simulink model "cantonisim_distributed_3pools"  (R2019b)
settings: Solver=VariableStepAuto  StartTime=0.0  StopTime=800  FixedStep=1  RelTol=1e-3
InitFcn:
  | ini_cantonisim_distributed
values from neighbouring files (symbols this model uses):
  alpha = [6492, 2478, 6084, 5658, 7650, 6492]    [cantoni_2008_values.m]    (also in cantoni_LMI.m = [6492, 2478, 6084, 5658, 7650]; distributed_workspace.mat = [6492 2478 6084 5658 7650])
  kappa = [1.69, 6.47, 2.37, 2.21, 1.68, 1.69]    [cantoni_2008_values.m]    (also in cantoni_LMI.m = [1.69, 6.47, 2.37, 2.21, 1.68]; distributed_workspace.mat = [1.69 6.47 2.37 2.21 1.68]; lab_setup_values.m = [0.3, 0.5, 0.3])
  phi = [113.64, 37.17, 86.96, 96.15, 113.64, 113.64]    [cantoni_2008_values.m]    (also in cantoni_LMI.m = [113.64, 37.17, 86.96, 96.15, 113.64]; distributed_workspace.mat = [113.64 37.17 86.96 96.15 113.64]; lab_setup_values.m = [10, 10, 10])
  rho = [9.97, 3.26, 7.60, 8.47, 9.97, 9.97]    [cantoni_2008_values.m]    (also in cantoni_LMI.m = [9.97, 3.26, 7.60, 8.47, 9.97]; distributed_workspace.mat = [9.97 3.26 7.6 8.47 9.97]; lab_setup_values.m = [0.1, 0.1, 0.1])
  tau = [4, 2, 4, 4, 6, 4]    [cantoni_2008_values.m]    (also in cantoni_LMI.m = [4, 2, 4, 4, 6]; distributed_workspace.mat = [4 2 4 4 6])
  w_n = zeros(1,length(phi_wave))    [cantoni_2008_values.m]    (also in cantoni_LMI.m; distributed_workspace.mat = [0.48005473176 1.05011972572 0.48005473176 0.48005473176 0.4)
  zeta = 0.0151    [distributed_workspace.mat]
undefined symbols (not defined in the file or in its folder): SA, SB, SC, SD
settings Model: Creator=Jacob  LastModifiedBy=bas
settings SolverCC: AlgebraicLoopSolver=LineSearch
settings ModelReferenceCC: ModelReferenceMinAlgLoopOccurrences=on
settings SFSimCC: CustomCodeUndefinedFunction=UseInterfaceOnly

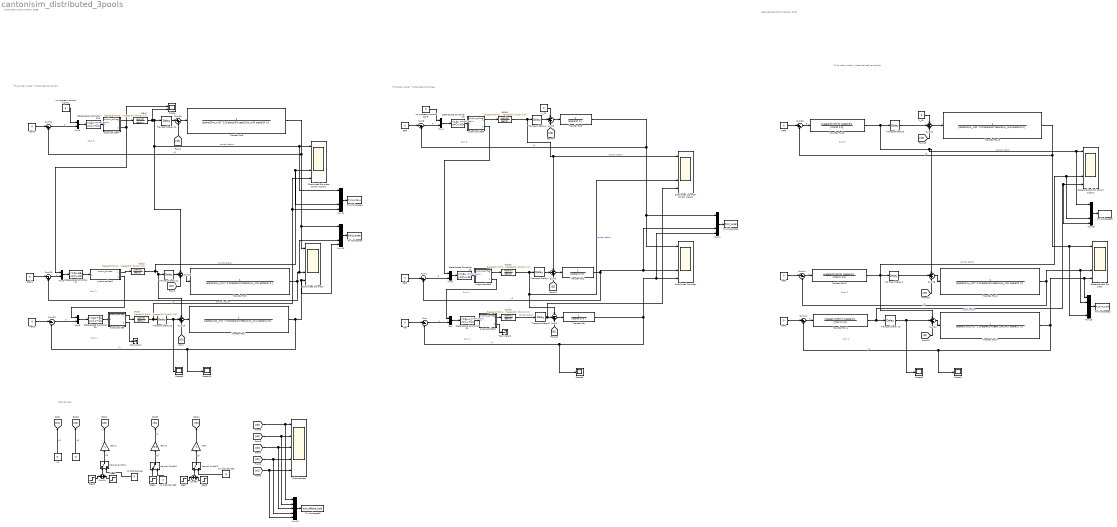
== system cantonisim_distributed_3pools ==
  note: Disturbances
  note: Decentralied Control Cantoni 2007
  note: Third order model + decentralized controllers
  note: First order model + distributed controllers
  note: Pool 1
  note: Distributed Control Cantoni 2008
  note: Pool 2
  note: Pool 5
  note: Pool 1
  note: Pool 5
  note: Pool 2
  note: Third order model + distributed controllers
  note: Pool 5
  note: Pool 1
  note: Pool 2
  " " : Constant  Value=0
  Decentralized 3rd control signals : Scope  NumInputPorts=5
  Decentralized 3rd order : Scope  NumInputPorts=5
  Distributed 1st order : Scope  NumInputPorts=5
  Distributed 1st order control signals : Scope  NumInputPorts=5
  Distributed 3rd order : Scope  NumInputPorts=5
  Distributed 3rd order control signals : Scope  NumInputPorts=5
  Disturbances : Scope  NumInputPorts=5
  Gain : Gain  Gain=-1
  Gain1 : Gain  Gain=-1
  Gain2 : Gain  Gain=-0.5
  Manual Switch1 : ManualSwitch
  Manual Switch2 : ManualSwitch
  Manual Switch3 : ManualSwitch
  Mux{,1,4..6,9} (6 alike) : Mux  Inputs=2
  Mux{10..15} (6 alike) : Mux  Inputs=5
  Ref{,1,4..6,9..11,14} (9 alike) : Constant  Value=0
  Scope : Scope  NumInputPorts=2
  Scope{3,5,7..8,10} (5 alike) : Scope
  State-Space Controller S1 : StateSpace  A=SA{1}  B=SB{1}  C=SC{1}  D=SD{1}  InitialCondition=0
  State-Space Controller S10 : StateSpace  A=SA{3}  B=SB{3}  C=SC{3}  D=SD{3}  InitialCondition=0
  State-Space Controller S2 : StateSpace  A=SA{2}  B=SB{2}  C=SC{2}  D=SD{2}  InitialCondition=0
  State-Space Controller S5 : StateSpace  A=SA{3}  B=SB{3}  C=SC{3}  D=SD{3}  InitialCondition=0
  State-Space Controller S6 : StateSpace  A=SA{1}  B=SB{1}  C=SC{1}  D=SD{1}  InitialCondition=0
  State-Space Controller S7 : StateSpace  A=SA{2}  B=SB{2}  C=SC{2}  D=SD{2}  InitialCondition=0
  Step1 : Step  Time=100  SampleTime=0
  Step5 : Step  Time=10  SampleTime=0
  Step6 : Step  Time=20  After=-1  SampleTime=0
  Step7 : Step  Time=100  SampleTime=0
  Step8 : Step  Time=150  After=-1  SampleTime=0
  Sum{,10,14,20} (4 alike) : Sum  Inputs=|+-
  Sum{1,3,9,12,15,21,23,26} (8 alike) : Sum  Inputs=-++
  Sum{2,8,25,31} (4 alike) : Sum  Inputs=|-+
  Sum22 : Sum  Inputs=|--
  Sum24 : Sum  Inputs=+|+
  Sum32 : Sum  Inputs=|++
  Sum33 : Sum  Inputs=+|+
  Terminator : Terminator
  Terminator1 : Terminator
  To Workspace : ToWorkspace  VariableName=third_order  SaveFormat=Structure With Time  SampleTime=-1
  To Workspace1 : ToWorkspace  VariableName=first_order  SaveFormat=Structure With Time  SampleTime=-1
  To Workspace2 : ToWorkspace  VariableName=dist_offtake_load  SaveFormat=Structure With Time  SampleTime=-1
  To Workspace3 : ToWorkspace  VariableName=PI_third_order  SaveFormat=Structure With Time  SampleTime=-1
  To Workspace4 : ToWorkspace  VariableName=third_order_u  SaveFormat=Structure With Time  SampleTime=-1
  To Workspace5 : ToWorkspace  VariableName=PI_third_order_u  SaveFormat=Structure With Time  SampleTime=-1
  Transfer Fcn : TransferFcn  Denominator=[alpha(1) 0 ]
  Transfer Fcn1 : TransferFcn  Denominator=[alpha(1)/w_n(1)^2 2*alpha(1)*zeta(1)/w_n(1) alpha(1) 0 ]
  Transfer Fcn10 : TransferFcn  Denominator=[alpha(1)/w_n(1)^2 2*alpha(1)*zeta(1)/w_n(1) alpha(1) 0 ]
  Transfer Fcn11 : TransferFcn  Numerator=[kappa(1)*phi(1) kappa(1)]  Denominator=[rho(1) 1 0]
  Transfer Fcn12 : TransferFcn  Denominator=[alpha(2)/w_n(2)^2 2*alpha(2)*zeta(2)/w_n(2) alpha(2) 0 ]
  Transfer Fcn13 : TransferFcn  Numerator=[kappa(2)*phi(2) kappa(2)]  Denominator=[rho(2) 1 0]
  Transfer Fcn18 : TransferFcn  Denominator=[alpha(3)/w_n(3)^2 2*alpha(3)*zeta(3)/w_n(3) alpha(3) 0 ]
  Transfer Fcn19 : TransferFcn  Numerator=[kappa(3)*phi(3) kappa(3)]  Denominator=[rho(3) 1 0]
  Transfer Fcn2 : TransferFcn  Denominator=[alpha(2) 0 ]
  Transfer Fcn3 : TransferFcn  Denominator=[alpha(2)/w_n(2)^2 2*alpha(2)*zeta(2)/w_n(2) alpha(2) 0 ]
  Transfer Fcn8 : TransferFcn  Denominator=[alpha(3) 0 ]
  Transfer Fcn9 : TransferFcn  Denominator=[alpha(3)/w_n(3)^2 2*alpha(3)*zeta(3)/w_n(3) alpha(3) 0 ]
  Transport Delay1 : TransportDelay  DelayTime=tau(2)
  Transport Delay10 : TransportDelay  DelayTime=tau(1)
  Transport Delay11 : TransportDelay  DelayTime=tau(2)
  Transport Delay14 : TransportDelay  DelayTime=tau(3)
  Transport Delay15 : TransportDelay  DelayTime=tau(1)
  Transport Delay4 : TransportDelay  DelayTime=tau(3)
  Transport Delay5 : TransportDelay  DelayTime=tau(1)
  Transport Delay6 : TransportDelay  DelayTime=tau(2)
  Transport Delay9 : TransportDelay  DelayTime=tau(3)
  V_N1 : Constant  Value=0
  V_N2 : Constant  Value=0
  W1(s) : TransferFcn  Numerator=[kappa(1)*phi(1) kappa(1)]  Denominator=[rho(1) 1 0]
  W1(s)1 : TransferFcn  Numerator=[kappa(1)*phi(1) kappa(1)]  Denominator=[rho(1) 1 0]
  W2(s) : TransferFcn  Numerator=[kappa(2)*phi(2) kappa(2)]  Denominator=[rho(2) 1 0]
  W2(s)1 : TransferFcn  Numerator=[kappa(2)*phi(2) kappa(2)]  Denominator=[rho(2) 1 0]
  W5(s) : TransferFcn  Numerator=[kappa(3)*phi(3) kappa(3)]  Denominator=[rho(3) 1 0]
  W5(s)1 : TransferFcn  Numerator=[kappa(3)*phi(3) kappa(3)]  Denominator=[rho(3) 1 0]
  no : Constant  Value=0
  no disturbance1 : Constant  Value=0
  no disturbance2 : Constant  Value=0
  no disturbance3 : Constant  Value=0
  no upstream control signal : Constant  Value=0
  no upstream control signal1 : Constant  Value=0
  output splitter{,1,4..5,8..9} (6 alike) : ModelReference  ModelNameDialog=output_splitter  SimulationMode=Normal  ModelReferenceVersion=1.52
  wires:
  W1(s)1/1 -> Transport Delay5/1  "control action"
  Sum/1 -> Mux/2  "e"
  Ref/1 -> Sum/1
  Transport Delay5/1 -> Distributed 1st order control signals/5, Sum1/2
  Sum1/1 -> Transfer Fcn/1
  [d1] -> Sum1/3
  Transport Delay1/1 -> Sum3/2
  Transfer Fcn2/1 -> Sum2/2, Mux11/4, Distributed 1st order/4  "y2"
  Sum3/1 -> Transfer Fcn2/1
  W2(s)1/1 -> Distributed 1st order control signals/4, Sum1/1, Transport Delay1/1  "control action"
  Sum2/1 -> Mux1/2  "e"
  [d2] -> Sum3/3
  Sum8/1 -> Mux4/2  "e"
  Sum9/1 -> Transfer Fcn8/1
  W5(s)1/1 -> Sum3/1, Distributed 1st order control signals/1, Transport Delay4/1  "control action"
  Transfer Fcn8/1 -> Mux11/1, Distributed 1st order/1, Sum8/2  "y5"
  Transport Delay4/1 -> Sum9/2
  V_N2/1 -> Sum9/1
  [d5] -> Sum9/3
  Transfer Fcn/1 -> Scope3/1, Sum/2, Mux11/5, Distributed 1st order/5  "y1"
  Ref1/1 -> Sum2/1
  Ref4/1 -> Sum8/1
  Transport Delay10/1 -> Scope5/1, Sum12/2
  Sum12/1 -> Transfer Fcn10/1
  Transport Delay9/1 -> Sum21/2
  V_N1/1 -> Sum21/1
  Transfer Fcn19/1 -> Sum15/1, Mux15/1, Decentralized 3rd control signals/1, Transport Delay9/1  "control action"
  [d1] -> Sum12/3
  Sum20/1 -> Transfer Fcn19/1  "e"
  [d5] -> Sum21/3
  Sum15/1 -> Transfer Fcn12/1
  Sum14/1 -> Transfer Fcn13/1  "e"
  Sum21/1 -> Transfer Fcn18/1
  Sum10/1 -> Transfer Fcn11/1  "e"
  Transport Delay6/1 -> Sum15/2
  Transfer Fcn13/1 -> Mux15/4, Decentralized 3rd control signals/4, Sum12/1, Transport Delay6/1  "control action"
  Ref6/1 -> Sum14/1
  Transfer Fcn12/1 -> Mux13/2, Decentralized 3rd order/4, Sum14/2  "y2"
  Ref9/1 -> Sum20/1
  [d2] -> Sum15/3
  Transfer Fcn10/1 -> Scope7/1, Sum10/2, Mux13/1, Decentralized 3rd order/5  "y1"
  Ref5/1 -> Sum10/1
  Transfer Fcn18/1 -> Sum20/2, Mux13/5, Decentralized 3rd order/1  "y5"
  Transfer Fcn11/1 -> Mux15/5, Decentralized 3rd control signals/5, Transport Delay10/1  "ontrol action"
  Mux/1 -> State-Space Controller S1/1
  Mux1/1 -> State-Space Controller S2/1
  Mux4/1 -> State-Space Controller S5/1
  no upstream control signal/1 -> Mux4/1
  Mux6/1 -> State-Space Controller S7/1
  Mux5/1 -> State-Space Controller S6/1
  [d2] -> Sum26/3
  Transfer Fcn3/1 -> Mux10/4, Distributed 3rd order/4, Sum25/2  "y2"
  Sum26/1 -> Transfer Fcn3/1
  Transport Delay15/1 -> Scope8/1, Sum23/2
  Sum22/1 -> Mux5/2  "e"
  Sum31/1 -> Mux9/2  "e"
  Transfer Fcn9/1 -> Sum31/2, Mux10/1, Distributed 3rd order/1  "y5"
  Transport Delay11/1 -> Sum26/2
  Mux9/1 -> State-Space Controller S10/1
  Transfer Fcn1/1 -> Scope10/1, Sum22/2, Mux10/5, Distributed 3rd order/5  "y1"
  W1(s)/1 -> Distributed 3rd order control signals/5, Mux14/5, Transport Delay15/1  "control action"
  W2(s)/1 -> Distributed 3rd order control signals/4, Mux14/4, Sum23/1, Transport Delay11/1  "control action"
  no upstream control signal1/1 -> Mux9/1
  Transport Delay14/1 -> Sum32/1
  Sum32/1 -> Transfer Fcn9/1
  Ref10/1 -> Sum22/1
  Ref11/1 -> Sum25/1
  Ref14/1 -> Sum31/1
  Sum23/1 -> Transfer Fcn1/1
  Sum25/1 -> Mux6/2  "e"
  [d1] -> Sum23/3
  no disturbance1/1 -> Manual Switch1/2
  Step5/1 -> Sum24/1
  Sum24/1 -> Manual Switch1/1
  Step6/1 -> Sum24/2
  Manual Switch1/1 -> Gain1/1  "d3"
  " "/1 -> [d2]  "d2"
  Gain2/1 -> [d4]  "d4"
  Manual Switch2/1 -> Gain/1  "d5"
  [d5] -> Sum32/2
  no/1 -> [d1]  "d1"
  Step8/1 -> Sum33/2
  Sum33/1 -> Manual Switch2/1
  Step7/1 -> Sum33/1
  no disturbance2/1 -> Manual Switch2/2
  [d3] -> Mux12/3, Disturbances/3
  [d1] -> Mux12/5, Disturbances/5
  [d5] -> Mux12/1, Disturbances/1
  [d2] -> Disturbances/4, Mux12/4
  [d4] -> Mux12/2, Disturbances/2
  State-Space Controller S6/1 -> output splitter/1
  State-Space Controller S7/1 -> output splitter1/1
  State-Space Controller S10/1 -> output splitter4/1  "control action"
  output splitter4/2 -> Mux6/1, Scope/1
  output splitter1/2 -> Mux5/1
  output splitter/1 -> W1(s)/1
  output splitter1/1 -> W2(s)/1
  output splitter4/1 -> W5(s)/1
  W5(s)/1 -> Scope/2, Sum26/1, Distributed 3rd order control signals/1, Mux14/1, Transport Delay14/1  "control action"
  Gain/1 -> [d5]
  Gain1/1 -> [d3]
  Manual Switch3/1 -> Gain2/1  "d5"
  no disturbance3/1 -> Manual Switch3/2
  Step1/1 -> Manual Switch3/1
  State-Space Controller S5/1 -> output splitter5/1  "control action"
  output splitter5/1 -> W5(s)1/1
  output splitter5/2 -> Mux1/1
  State-Space Controller S2/1 -> output splitter8/1  "control action"
  output splitter8/1 -> W2(s)1/1
  output splitter8/2 -> Mux/1
  State-Space Controller S1/1 -> output splitter9/1  "control action"
  output splitter9/1 -> W1(s)1/1
  Mux10/1 -> To Workspace/1
  Mux11/1 -> To Workspace1/1
  Mux12/1 -> To Workspace2/1
  Mux13/1 -> To Workspace3/1
  Mux14/1 -> To Workspace4/1
  Mux15/1 -> To Workspace5/1
  output splitter/2 -> Terminator/1
  output splitter9/2 -> Terminator1/1
